simulink model "arm_sim"  (R2016b)
settings: Solver=ode45  StartTime=0.0  StopTime=50  RelTol=1e-3  EnableMultiTasking=on
InitFcn:
  | addpath ./..
  | arm_param
  | armParamHW8
undefined symbols (not defined in the file): P
settings Model: Creator=beard  LastModifiedBy=beard
settings DataIOCC: LimitDataPoints=on  SaveFormat=Array  SignalLoggingSaveFormat=ModelDataLogs
settings OptimizationCC: ExpressionDepthLimit=2147483647  InitFltsAndDblsToZero=on  LifeSpan=inf
settings DebuggingCC: UnderspecifiedInitializationDetection=Classic  MergeDetectMultiDrivingBlocksExec=none  SolverPrmCheckMsg=warning  FcnCallInpInsideContextMsg=warning  StateNameClashWarn=warning  SFUnexpectedBacktrackingDiag=warning  SFNoUnconditionalDefaultTransitionDiag=warning  SFExecutionAtInitializationDiag=none
settings HardwareCC: ProdBitPerPointer=32  ProdBitPerSizeT=32  ProdBitPerPtrDiffT=32  ProdLargestAtomicFloat=None  ProdIntDivRoundTo=Undefined  ProdEndianess=Unspecified  ProdWordSize=32  ProdHWDeviceType=32-bit Generic
settings ModelReferenceCC: PropagateSignalLabelsOutOfModel=off
settings GRTTargetCC: TargetLangStandard=C89/C90 (ANSI)  GeneratePreprocessorConditionals=Disable all  CombineOutputUpdateFcns=off  GRTInterface=on
settings ConfigComp: CovMetricSettings=dw  CovHtmlReporting=on  CovSaveCumulativeToWorkspaceVar=on  CovSaveSingleToWorkspaceVar=on  CovExternalEMLEnable=off

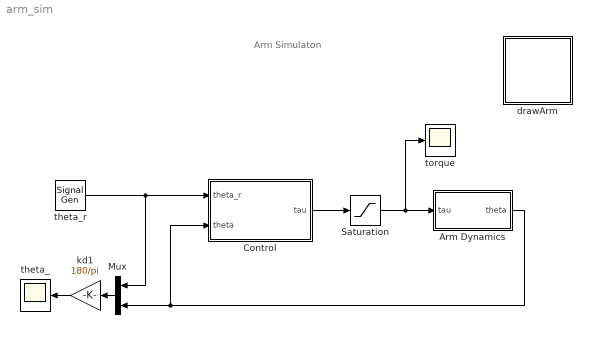
== system arm_sim ==
  note: Arm Simulaton
  "Arm Dynamics " : Subsystem
  Control : Subsystem
  Mux : Mux  Inputs=2
  Saturation : Saturate  UpperLimit=P.tau_max  LowerLimit=-P.tau_max
  drawArm : Subsystem
      mask Display: image(imread('tv.jpg'))
  kd1 : Gain  Gain=180/pi
  theta_ : Scope
  theta_r : SignalGenerator  WaveForm=square  Amplitude=25*pi/180  Frequency=.05
  torque : Scope
  wires:
  theta_r/1 -> Control/1(theta_r), Mux/1
  Mux/1 -> kd1/1
  kd1/1 -> theta_/1
  Control/1(tau) -> Saturation/1
  Saturation/1 -> torque/1, "Arm Dynamics "/1(tau)
  "Arm Dynamics "/1("theta ") -> Control/2(theta), Mux/2

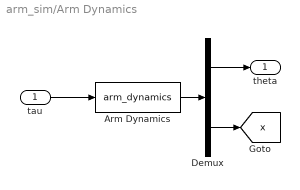
== system arm_sim/Arm Dynamics  ==
  tau : Inport
  Arm Dynamics : S-Function  FunctionName=arm_dynamics  Parameters=P  SFunctionDeploymentMode=off  EnableBusSupport=off
  Demux : Demux  Outputs=[1;2]
  "theta " : Outport
  tag scope: x=global
  wires:
  tau/1 -> Arm Dynamics/1
  Demux/1 -> "theta "/1
  Demux/2 -> [x]
  Arm Dynamics/1 -> Demux/1

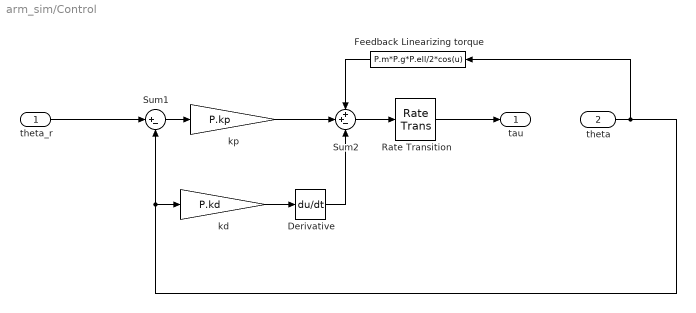
== system arm_sim/Control ==
  theta_r : Inport
  theta : Inport  Port=2
  Derivative : Derivative  CoefficientInTFapproximation=P.sigma
  Feedback Linearizing torque : Fcn  Expr=P.m*P.g*P.ell/2*cos(u)
  Rate Transition : RateTransition  OutPortSampleTime=P.Ts
  Sum1 : Sum  Inputs=|+-
  Sum2 : Sum  Inputs=++-
  kd : Gain  Gain=P.kd
  kp : Gain  Gain=P.kp
  tau : Outport
  wires:
  Rate Transition/1 -> tau/1
  theta_r/1 -> Sum1/1
  Sum2/1 -> Rate Transition/1
  Sum1/1 -> kp/1
  kp/1 -> Sum2/2
  kd/1 -> Derivative/1
  Derivative/1 -> Sum2/3
  Feedback Linearizing torque/1 -> Sum2/1
  theta/1 -> Feedback Linearizing torque/1, kd/1, Sum1/2

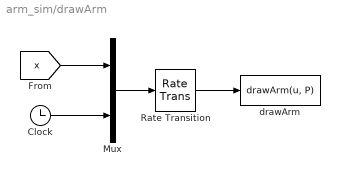
== system arm_sim/drawArm ==
  Clock : Clock
  Mux : Mux  Inputs=2
  Rate Transition : RateTransition  OutPortSampleTime=P.t_plot
  drawArm : MATLABFcn  MATLABFcn=drawArm(u, P)  OutputDimensions=0
  wires:
  Rate Transition/1 -> drawArm/1
  Mux/1 -> Rate Transition/1
  Clock/1 -> Mux/2
  [x] -> Mux/1
